simulink model "kontrollubuck"  (R2014a)
settings: Solver=ode45  StartTime=0.0  StopTime=0.0012  RelTol=1e-3
values from neighbouring files (symbols this model uses):
  C = 470e-6    (= 0.00047)    [denemefonk.m]    (also in fa.m)
  ki = BestSol.Position(2)    [fa.m]
  kp = BestSol.Position(1)    [fa.m]
  L = 300e-6    (= 0.0003)    [denemefonk.m]    (also in fa.m)
  ts = 10e-6    (= 1e-05)    [denemefonk.m]    (also in fa.m)
undefined symbols (not defined in the file or in its folder): rc, rl
libraries: powerlib x23
settings Model: Creator=ahilem  LastModifiedBy=ahilem

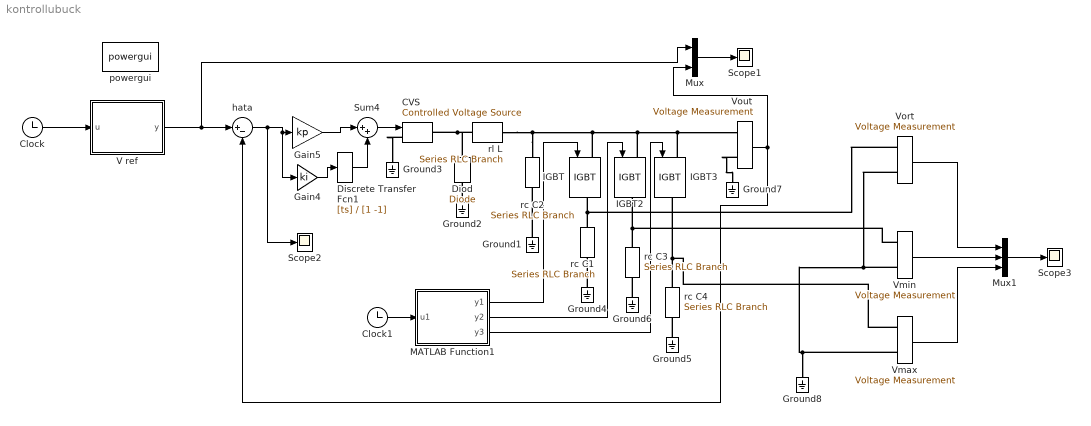
== system kontrollubuck ==
  CVS : powerlib/Electrical Sources/Controlled Voltage Source  Initialize=on  Source_Type=DC  Amplitude=0  Phase=0  Frequency=0  Measurements=None
  Clock : Clock
  Clock1 : Clock
  Diod : powerlib/Power Electronics/Diode  Ron=0.001  Lon=0  Vf=0.8  IC=0  UseSnubber=off  Rs=500  Cs=250e-9  Measurements=off
  Discrete Transfer Fcn1 : DiscreteTransferFcn  Numerator=[ts]  Denominator=[1 -1]  InitialStates=[0]  SampleTime=ts
  Gain4 : Gain  Gain=ki
  Gain5 : Gain  Gain=kp
  Ground{1..8} (8 alike) : powerlib/Elements/Ground  LConnTagsString=a
  IGBT : powerlib/Power Electronics/IGBT  Ron=0.001  Lon=0  Vf=1  Tf=1e-6  Tt=2e-6  IC=0  Rs=1e5  Cs=inf  Measurements=off
  IGBT2 : powerlib/Power Electronics/IGBT  Ron=0.001  Lon=0  Vf=1  Tf=1e-6  Tt=2e-6  IC=0  Rs=1e5  Cs=inf  Measurements=off
  IGBT3 : powerlib/Power Electronics/IGBT  Ron=0.001  Lon=0  Vf=1  Tf=1e-6  Tt=2e-6  IC=0  Rs=1e5  Cs=inf  Measurements=off
  MATLAB Function1 : MATLAB Function  TreatAsAtomicUnit=on
  Mux : Mux  Inputs=2
  Mux1 : Mux  Inputs=3
  Scope1 : Scope
      settings: ShowLegends=on  YMin=0  YMax=90
  Scope2 : Scope
      settings: ShowLegends=on  YMin=0  YMax=90
  Scope3 : Scope
      settings: ShowLegends=on  YMin=0  YMax=90  SaveName=ScopeData2
  Sum4 : Sum  Inputs=|++
  V ref : MATLAB Function  TreatAsAtomicUnit=on
  Vmax : powerlib/Measurements/Voltage Measurement  PhasorSimulation=off  OutputType=Complex  PSBequivalent=0
  Vmin : powerlib/Measurements/Voltage Measurement  PhasorSimulation=off  OutputType=Complex  PSBequivalent=0
  Vort : powerlib/Measurements/Voltage Measurement  PhasorSimulation=off  OutputType=Complex  PSBequivalent=0
  Vout : powerlib/Measurements/Voltage Measurement  PhasorSimulation=off  OutputType=Complex  PSBequivalent=0
  hata : Sum  Inputs=|+-
  powergui : powerlib/powergui  Priority=1  SimulationMode=Discrete  SolverType=Tustin  SampleTime=1e-6  frequency=60  SPID=off  DisableSnubberDevices=off  DisableRonSwitches=off  DisableVfSwitches=off  SwTol=0  Interpol=off  DisplayEquations=off  Ts=0  methode=off  frequencyindice=0  Pbase=100e6  ErrMax=1e-4  Iterations=50  UnitsV=kV  UnitsW=MW  FunctionMessages=off  echomessages=off  HookPort=off  EnableUseOfTLC=off  x0status=zero  RestoreLinks=warning  ResistiveCurrentMeasurement=off  Frange=[0:2:500]  Ylog=off  Xlog=on  ShowGrid=off  save=off  variable=ZData  structure=0  ZoomFFT=off  StartTime=0.0  cycles=1  DisplayStyle=1  fundamental=60  FreqAxis=off  MaxFrequency=1000  frequencyindicesteady=1  RmsSteady=1  display=off
  rc C1 : powerlib/Elements/Series RLC Branch  LConnTagsString=__new0  RConnTagsString=__new0  BranchType=R  Resistance=4.8  Inductance=1e-3  SetiL0=off  InitialCurrent=0  Capacitance=C  Setx0=off  InitialVoltage=0  Measurements=None
  rc C2 : powerlib/Elements/Series RLC Branch  LConnTagsString=__new0  RConnTagsString=__new0  BranchType=RC  Resistance=rc  Inductance=1e-3  SetiL0=off  InitialCurrent=0  Capacitance=C  Setx0=off  InitialVoltage=0  Measurements=None
  rc C3 : powerlib/Elements/Series RLC Branch  LConnTagsString=__new0  RConnTagsString=__new0  BranchType=R  Resistance=240  Inductance=1e-3  SetiL0=off  InitialCurrent=0  Capacitance=C  Setx0=off  InitialVoltage=0  Measurements=None
  rc C4 : powerlib/Elements/Series RLC Branch  LConnTagsString=__new0  RConnTagsString=__new0  BranchType=R  Resistance=2.4  Inductance=1e-3  SetiL0=off  InitialCurrent=0  Capacitance=C  Setx0=off  InitialVoltage=0  Measurements=None
  rl L : powerlib/Elements/Series RLC Branch  LConnTagsString=__new0  RConnTagsString=__new0  BranchType=RL  Resistance=rl  Inductance=L  SetiL0=off  InitialCurrent=0  Capacitance=1e-6  Setx0=off  InitialVoltage=0  Measurements=None
  wires:
  Sum4/1 -> CVS/1
  hata/1 -> Scope2/1, Gain4/1, Gain5/1
  Gain5/1 -> Sum4/1
  Discrete Transfer Fcn1/1 -> Sum4/2
  Gain4/1 -> Discrete Transfer Fcn1/1
  Vout/1 -> Mux/2, hata/2
  Clock/1 -> V ref/1(u)
  V ref/1(y) -> Mux/1, hata/1
  Mux/1 -> Scope1/1
  Clock1/1 -> MATLAB Function1/1(u1)
  MATLAB Function1/2(y2) -> IGBT2/1
  MATLAB Function1/3(y3) -> IGBT3/1
  MATLAB Function1/1(y1) -> IGBT/1
  Mux1/1 -> Scope3/1
  Vmin/1 -> Mux1/2
  Vort/1 -> Mux1/1
  Vmax/1 -> Mux1/3
  connections:
  CVS/LConn1 -- Ground3/LConn1
  Ground2/LConn1 -- Diod/LConn1
  Diod/RConn1 -- rl L/LConn1 -- CVS/RConn1
  Ground1/LConn1 -- rc C2/RConn1
  Ground4/LConn1 -- rc C1/RConn1
  Ground6/LConn1 -- rc C3/RConn1
  rc C3/LConn1 -- Vmin/LConn1 -- IGBT2/RConn1
  Ground5/LConn1 -- rc C4/RConn1
  rc C4/LConn1 -- IGBT3/RConn1 -- Vmax/LConn1
  rc C1/LConn1 -- Vort/LConn1 -- IGBT/RConn1
  rc C2/LConn1 -- IGBT2/LConn1 -- IGBT3/LConn1 -- Vout/LConn1 -- IGBT/LConn1 -- rl L/RConn1
  Vout/LConn2 -- Ground7/LConn1
  Vort/LConn2 -- Vmax/LConn2 -- Ground8/LConn1 -- Vmin/LConn2

== matlab function kontrollubuck/MATLAB Function1 ==
  data: u1 input; y1 output; y2 output; y3 output
function [y1,y2,y3]  = fcn(u1)
%#codegen

if u1<200e-6
  y1=1;
  y2=0;
  y3=0;
elseif u1<600e-6
  y1=0;
  y2=1;
  y3=0;
else
    y1=0;
  y2=0;
  y3=1;
end

== matlab function kontrollubuck/V ref ==
  data: u input; y output
function y = fcn(u)

if u<400e-6
    y=12;
elseif u<800e-6
  y=5;  
else
   y=12; 
end
